simulink model "AdmittanceSimulationFirstOrderFilter"  (R2018b)
settings: Solver=ode23  StartTime=0.0  StopTime=60  RelTol=1e-3
values from neighbouring files (symbols this model uses):
  N = zeros(3, 7)    [InverseDynamic.m]
  s = (InverseDynamic(jointVelocity,joint ,a) - C)    [ForwardDynamicSolver.m]
undefined symbols (not defined in the file or in its folder): X, Y, Z
libraries: sm_lib x60, nesl_utility x36
(part 2 of 2)

== system AdmittanceSimulationFirstOrderFilter/Robot/DynamicModel/wrist_upper_link ==
  Inertia : sm_lib/Body Elements/Inertia  InertiaType=Custom  Mass=0.1956991  MassUnits=kg  CenterOfMass=[0, 0, 0]  CenterOfMassUnits=m  MomentsOfInertia=[7.035e-05, 0.0001151, 0.00013235]  MomentsOfInertiaUnits=kg*m^2  ProductsOfInertia=[0, 0, -1.5e-06]  ProductsOfInertiaUnits=kg*m^2  GraphicType=None  MarkerShape=Inertia  MarkerSize=20  GraphicVisPropType=SimpleVisualProperties  GraphicDiffuseColor=[0.5 0.5 0.5]  GraphicSpecularColor=[0.5 0.5 0.5 1.0]  GraphicAmbientColor=[0.15 0.15 0.15 1.0]  GraphicEmissiveColor=[0.0 0.0 0.0 1.0]  GraphicShininess=75  GraphicOpacity=1.0
  InertiaOriginTransform : sm_lib/Frames and Transforms/Rigid Transform  TranslationMethod=Cartesian  TranslationStandardOffset=0  TranslationLengthUnit=m  TranslationStandardAxis=+Z  TranslationCartesianOffset=[-0.03893593, 0.00017228, -2.84e-06]  TranslationROffset=0  TranslationROffsetUnits=m  TranslationZOffset=0  TranslationZOffsetUnits=m  TranslationThetaOffset=0  TranslationThetaOffsetUnits=deg  RotationMethod=RotationSequence  RotationAngleUnits=deg  RotationStandardAxis=+Z  RotationAngle=0.0  RotationArbitraryAxis=[0 0 1]  FollAlignAxisA=+X  BaseAlignAxisA=+Y  FollAlignAxisB=+Y  BaseAlignAxisB=+Z  RotationSequenceAxes=BaseAxes  RotationSequence=XYZ  RotationSequenceAngles=[0, 0, 0]  RotationSequenceAnglesUnits=rad  RotationMatrix=[1 0 0; 0 1 0; 0 0 1]
  ReferenceFrame : sm_lib/Frames and Transforms/Reference Frame
  wrist_pitch_joint_AxisTransform : sm_lib/Frames and Transforms/Rigid Transform  TranslationMethod=Cartesian  TranslationStandardOffset=0  TranslationLengthUnit=m  TranslationStandardAxis=+Z  TranslationCartesianOffset=[0, 0, 0]  TranslationROffset=0  TranslationROffsetUnits=m  TranslationZOffset=0  TranslationZOffsetUnits=m  TranslationThetaOffset=0  TranslationThetaOffsetUnits=deg  RotationMethod=ArbitraryAxis  RotationAngleUnits=rad  RotationStandardAxis=+Z  RotationAngle=0  RotationArbitraryAxis=[1, 0, 0]  FollAlignAxisA=+X  BaseAlignAxisA=+Y  FollAlignAxisB=+Y  BaseAlignAxisB=+Z  RotationSequenceAxes=FollowerAxes  RotationSequence=XYX  RotationSequenceAngles=[0 0 0]  RotationSequenceAnglesUnits=deg  RotationMatrix=[1 0 0; 0 1 0; 0 0 1]
  wrist_pitch_joint_OriginTransform : sm_lib/Frames and Transforms/Rigid Transform  TranslationMethod=Cartesian  TranslationStandardOffset=0  TranslationLengthUnit=m  TranslationStandardAxis=+Z  TranslationCartesianOffset=[-0.0606, 0, 0]  TranslationROffset=0  TranslationROffsetUnits=m  TranslationZOffset=0  TranslationZOffsetUnits=m  TranslationThetaOffset=0  TranslationThetaOffsetUnits=deg  RotationMethod=RotationSequence  RotationAngleUnits=deg  RotationStandardAxis=+Z  RotationAngle=0.0  RotationArbitraryAxis=[0 0 1]  FollAlignAxisA=+X  BaseAlignAxisA=+Y  FollAlignAxisB=+Y  BaseAlignAxisB=+Z  RotationSequenceAxes=BaseAxes  RotationSequence=XYZ  RotationSequenceAngles=[1.5708, -1.5708, 0]  RotationSequenceAnglesUnits=rad  RotationMatrix=[1 0 0; 0 1 0; 0 0 1]
  F : PMIOPort  Side=Left
  F1 : PMIOPort  Port=2  Side=Right
  connections:
  Inertia/RConn1 -- InertiaOriginTransform/RConn1
  InertiaOriginTransform/LConn1 -- ReferenceFrame/RConn1 -- wrist_pitch_joint_OriginTransform/LConn1 -- F/RConn1
  wrist_pitch_joint_AxisTransform/RConn1 -- F1/RConn1
  wrist_pitch_joint_AxisTransform/LConn1 -- wrist_pitch_joint_OriginTransform/RConn1

== matlab function AdmittanceSimulationFirstOrderFilter/MATLAB Function3 ==
  data: jointAngle input; tau output
function tau = GravityModel(jointAngle)
    robotParam = RobotParam;
    v_dot  = zeros(3, 8);
    R      = zeros(3, 3, 8);
    P      = zeros(3, 8);
    Pc     = zeros(3, 7);
    F      = zeros(3, 7);
    f      = zeros(3, 8);
    n      = zeros(3, 8);
    tau    = zeros(1, 7);
        
    v_dot(:, 1) = [0; 0; -9.81];
    
    for i = 1:(robotParam.mActuatorCount)
        R(:,:,i) = tform2rotm(robotParam.mJointReferentiel(:, :, i)) * (rotz(jointAngle(i) + robotParam.mJointOffset(i)));
        P(:, i)  = tform2trvec(robotParam.mJointReferentiel(:, :, i));
        Pc(:, i) = robotParam.mLinkCenterOfMass(:, i);
    end
    
    R(:,:, robotParam.mActuatorCount + 1) = zeros(3,3);
    P(:, robotParam.mActuatorCount + 1)   = [0;0;0];
    
    for i = 2:(robotParam.mActuatorCount + 1)
        v_dot(:, i) = R(:, :, i - 1)' * v_dot(:, i - 1);
        F(:, i - 1) = robotParam.mLinkMass(i - 1) * v_dot(:, i);
    end
    
    f(:, robotParam.mActuatorCount + 1) = [0; 0; 0];
    n(:, robotParam.mActuatorCount + 1) = [0; 0; 0];
    
    for i = (robotParam.mActuatorCount):-1:1
        f(:, i)   = R(:, :, i + 1) * f(:, i + 1) + F(:, i);
        n(:, i)   = R(:, :, i + 1) * n(:, i + 1) + cross(Pc(:, i), F(:, i)) + cross(P(:, i + 1), R(:, :, i + 1) * f(:, i + 1));
        tau(i)    = n(3,i);
    end     
end
